simulink model "origin_simulink"  (R2021b)
settings: Solver=VariableStepAuto  StartTime=0.0  StopTime=10  RelTol=1e-3
libraries: fuzblock x1, slpidlib x1
settings Model: Creator=lanzer  LastModifiedBy=lanzer

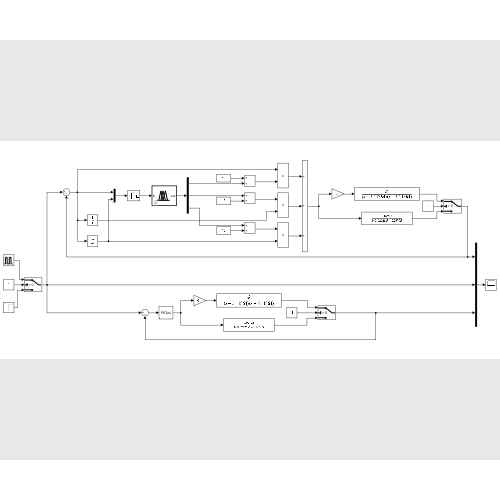
[thumbnail: Simulink's stored preview of the top-level diagram]
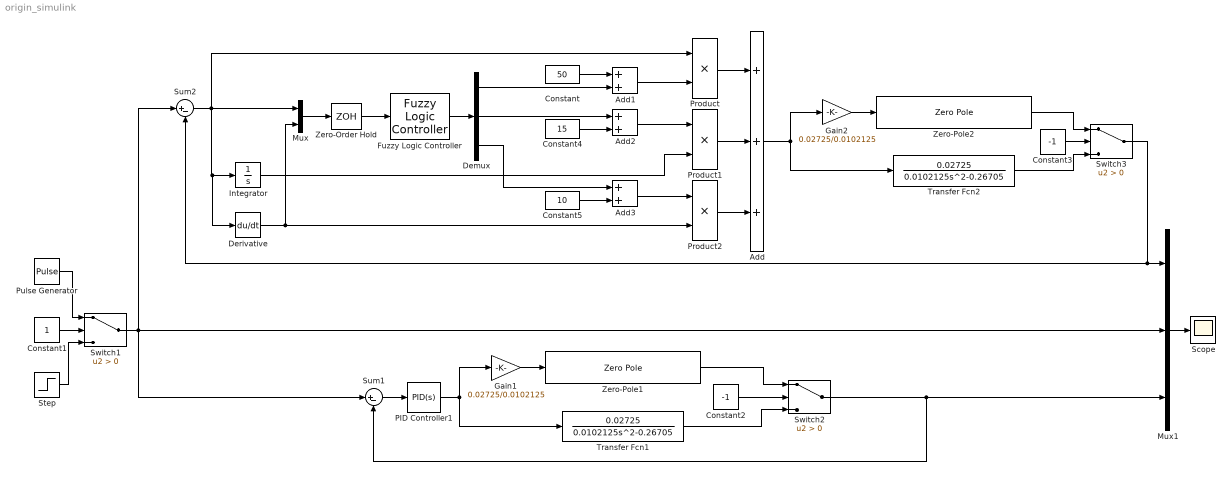
== system origin_simulink ==
  Add : Sum  Inputs=+++
  Add1 : Sum
  Add2 : Sum
  Add3 : Sum
  Constant : Constant  Value=50
  Constant1 : Constant
  Constant2 : Constant  Value=-1
  Constant3 : Constant  Value=-1
  Constant4 : Constant  Value=15
  Constant5 : Constant  Value=10
  Demux : Demux  Outputs=3
  Derivative : Derivative
  Fuzzy Logic Controller : fuzblock/Fuzzy Logic  Controller  FIS='FuzzyPID.fis'  OutputSampleNumber=101  DataType=double  FuzzifiedInputs=off  RuleFiringStrengths=off  RuleOutputs=off  AggregatedOutputs=off  SimulateUsing=Interpreted execution  OutOfRangeInputValueMessage=warning  NoRuleFiredMessage=warning  EmptyOutputFuzzySetMessage=warning
  Gain1 : Gain  Gain=0.02725/0.0102125
  Gain2 : Gain  Gain=0.02725/0.0102125
  Integrator : Integrator
  Mux : Mux  Inputs=2
  Mux1 : Mux  Inputs=3
  PID Controller1 : slpidlib/PID Controller  Controller=PID  Form=Parallel  TimeDomain=Continuous-time  UseExternalTs=off  SampleTime=-1  IntegratorMethod=Forward Euler  FilterMethod=Forward Euler  ControllerParametersSource=internal  P=50  I=15  D=10  UseFilter=on  N=100  TunerSelectOption=Transfer Function Based (PID Tuner App)  InitialConditionSource=internal  InitialConditionForIntegrator=0  InitialConditionForFilter=0  DifferentiatorICPrevScaledInput=0  ExternalReset=none  TrackingMode=off  Kt=1  LimitOutput=off  SatLimitsSource=internal  UpperSaturationLimit=inf  LowerSaturationLimit=-inf  LinearizeAsGain=on  AntiWindupMode=none  Kb=1  POutMin=[]  POutMax=[]  IOutMin=[]  IOutMax=[]  DOutMin=[]  DOutMax=[]  NOutMin=[]  NOutMax=[]  SumOutMin=[]  SumOutMax=[]  SaturationOutMin=[]  SaturationOutMax=[]  PParamMin=[]  PParamMax=[]  IParamMin=[]  IParamMax=[]  DParamMin=[]  DParamMax=[]  NParamMin=[]  NParamMax=[]  KbParamMin=[]  KbParamMax=[]  KtParamMin=[]  KtParamMax=[]  KbOutMin=[]  KbOutMax=[]  KtOutMin=[]  KtOutMax=[]  IntegratorOutMin=[]  IntegratorOutMax=[]  FilterOutMin=[]  FilterOutMax=[]  SumI1OutMin=[]  SumI1OutMax=[]  SumI2OutMin=[]  SumI2OutMax=[]  SumI3OutMin=[]  SumI3OutMax=[]  SumI4OutMin=[]  SumI4OutMax=[]  SumDOutMin=[]  SumDOutMax=[]  DifferentiatorOutMin=[]  DifferentiatorOutMax=[]  FilterDiffOutCoefMin=[]  FilterDiffOutCoefMax=[]  ReciprocalOutMin=[]  ReciprocalOutMax=[]  SumDenOutMin=[]  SumDenOutMax=[]  SumNumOutMin=[]  SumNumOutMax=[]  DivideOutMin=[]  DivideOutMax=[]  UdiffTsProdOutMin=[]  UdiffTsProdOutMax=[]  NTsProdOutMin=[]  NTsProdOutMax=[]  UintegralTsProdOutMin=[]  UintegralTsProdOutMax=[]  UngainTsProdOutMin=[]  UngainTsProdOutMax=[]  IntegratorContinuousStateAttributes=''  IntegratorStateMustResolveToSignalObject=off  IntegratorRTWStateStorageClass=Auto  FilterContinuousStateAttributes=''  FilterStateMustResolveToSignalObject=off  FilterRTWStateStorageClass=Auto  ParallelPVariant=InternalParameters  IdealPVariant=Disabled  IVariant=InternalParameters  DVariant=InternalParameters  IntegratorVariant=Continuous  SatVariant=Disabled  AWVariant=Passthrough  PCopyVariant=Disabled  TRVariant=Disabled  FdbkBlocksVariant=Forward  IdealPFdbkVariant=Disabled  SatFdbkVariant=Disabled  DerivativeFilterVariant=ContFilter  NVariant=InternalParameters  NCopyVariant=Disabled  FilterICVariant=InternalICsFilter  IntegratorICVariant=InternalICs  ExternalResetVariant=Disabled  TRSumVariant=Passthrough  SumFdbkVariant=Disabled  SumVariant=Sum_PID  TsampFilterVariant=InternalTs  TsampNgainVariant=Passthrough  TsampIntegralVariant=Passthrough  ExternalSaturationOutDataTypeStr=Inherit: Same as second input
  Product : Product
  Product1 : Product
  Product2 : Product
  Pulse Generator : DiscretePulseGenerator  PulseType=Time based  Period=4  PulseWidth=50
  Scope : Scope
  Step : Step  SampleTime=0
  Sum1 : Sum  Inputs=|+-
  Sum2 : Sum  Inputs=|+-
  Switch1 : Switch  Criteria=u2 > Threshold
  Switch2 : Switch  Criteria=u2 > Threshold
  Switch3 : Switch  Criteria=u2 > Threshold
  Transfer Fcn1 : TransferFcn  Numerator=[0.02725]  Denominator=[0.0102125 0 -0.26705]
  Transfer Fcn2 : TransferFcn  Numerator=[0.02725]  Denominator=[0.0102125 0 -0.26705]
  Zero-Order Hold : ZeroOrderHold  SampleTime=-1
  Zero-Pole1 : ZeroPole  Zeros=[0 0]  Poles=[5.11364 -5.11364]
  Zero-Pole2 : ZeroPole  Zeros=[0 0]  Poles=[5.11364 -5.11364]
  wires:
  PID Controller1/1 -> Transfer Fcn1/1, Gain1/1
  Transfer Fcn1/1 -> Switch2/3
  Zero-Pole1/1 -> Switch2/1
  Gain1/1 -> Zero-Pole1/1
  Constant2/1 -> Switch2/2
  Sum1/1 -> PID Controller1/1
  Constant3/1 -> Switch3/2
  Zero-Pole2/1 -> Switch3/1
  Transfer Fcn2/1 -> Switch3/3
  Gain2/1 -> Zero-Pole2/1
  Add/1 -> Transfer Fcn2/1, Gain2/1
  Product/1 -> Add/1
  Add1/1 -> Product/2
  Add2/1 -> Product1/1
  Add3/1 -> Product2/1
  Demux/1 -> Add1/2
  Demux/2 -> Add2/1
  Demux/3 -> Add3/1
  Fuzzy Logic Controller/1 -> Demux/1
  Mux/1 -> Zero-Order Hold/1
  Zero-Order Hold/1 -> Fuzzy Logic Controller/1
  Derivative/1 -> Mux/2, Product2/2
  Integrator/1 -> Product1/2
  Sum2/1 -> Product/1, Derivative/1, Integrator/1, Mux/1
  Pulse Generator/1 -> Switch1/1
  Constant1/1 -> Switch1/2
  Step/1 -> Switch1/3
  Switch1/1 -> Sum1/1, Sum2/1, Mux1/2
  Switch3/1 -> Mux1/1, Sum2/2
  Switch2/1 -> Sum1/2, Mux1/3
  Product1/1 -> Add/2
  Product2/1 -> Add/3
  Mux1/1 -> Scope/1
  Constant5/1 -> Add3/2
  Constant4/1 -> Add2/2
  Constant/1 -> Add1/1
